simulink model "nxtracer"  (Simulink 6.4)
settings: Solver=ode4  StartTime=0.0  StopTime=inf  FixedStep=Ts  RelTol=1e-3
PreLoadFcn:
  | param;
values from neighbouring files (symbols this model uses):
  CAMERA_POS = [100 100]    [param.m]
  Cm = 9.00e-6    (= 9e-06)    [param.m]
  Cw = 9.00e-4    (= 0.0009)    [param.m]
  Dx = 1e-3    (= 0.001)    [param.m]
  Dzz = 1e-6    (= 1e-06)    [param.m]
  e = -0.2    [param.m]
  J = M*(W/2)^2    (= 0.004096)    [param.m]
  Jm = 0.5e-7    (= 5e-08)    [param.m]
  Jw = 20.0e-7    (= 2e-06)    [param.m]
  Kb = 0.022    [param.m]
  Kt = 0.022    [param.m]
  LENGTH = 20    [param.m]
  LENGTH1 = 12    [param.m]
  LENGTH2 = 16    [param.m]
  LINE_MAP = ~(TRACK_MAP - LINE)    [param.m]
  Lm = 1.4e-3    (= 0.0014)    [param.m]
  M = 0.64    [param.m]
  n = 24    [param.m]
  Rm = 1.0    (= 1)    [param.m]
  Rw = 0.056/2    (= 0.028)    [param.m]
  START_POS = [148 100]    [param.m]
  TRACK_MAP = double(imread('track.bmp'))    [param.m]
  Ts = 0.0001    [param.m]
  W = 0.16    [param.m]
  WALL_MAP = ~(TRACK_MAP - WALL)    [param.m]
  WIDTH = 16    [param.m]
  WIDTH1 = 12    [param.m]
undefined symbols (not defined in the file or in its folder): clearNXTSignalObjects, DiscIntNeverNeededParam
libraries: simulink x12, vrlib x1, ecrobot_nxt_lib x1
(part 2 of 3)

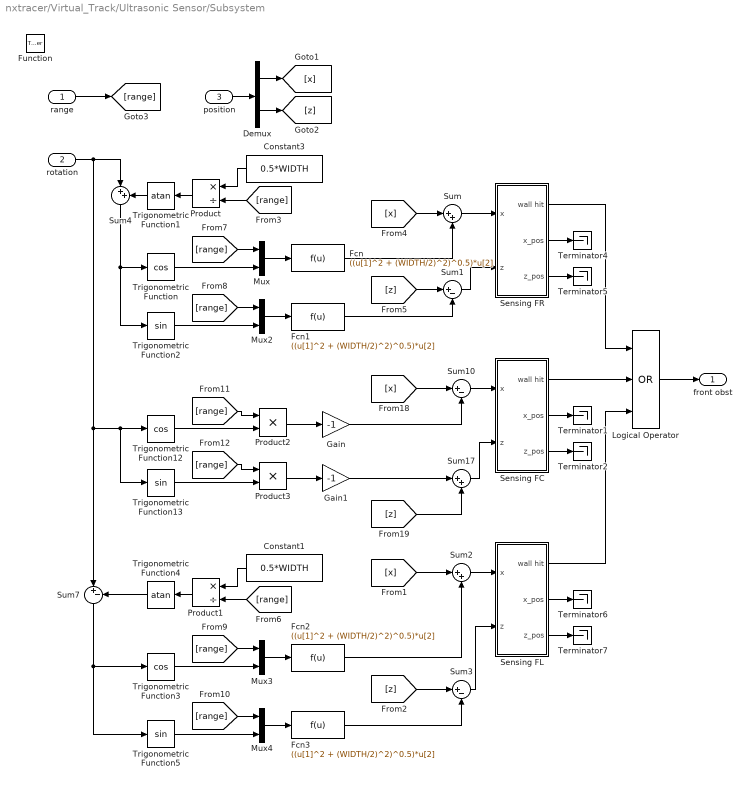
== system nxtracer/Virtual_Track/Ultrasonic Sensor/Subsystem ==
  range : Inport
  rotation : Inport  Port=2
  position : Inport  Port=3
  Function : TriggerPort  TriggerType=function-call
  Constant1 : Constant  Orientation=left  Value=0.5*WIDTH  OutDataType=sfix(16)  ConRadixGroup=Use specified scaling  OutScaling=2^0  SampleTime=inf  FramePeriod=inf
  Constant3 : Constant  Orientation=left  Value=0.5*WIDTH  OutDataType=sfix(16)  ConRadixGroup=Use specified scaling  OutScaling=2^0  SampleTime=inf  FramePeriod=inf
  Demux : Demux  Outputs=2
  Fcn{,1..3} (4 alike) : Fcn  Expr=((u[1]^2 + (WIDTH/2)^2)^0.5)*u[2]
  Gain : Gain  Gain=-1
  Gain1 : Gain  Gain=-1
  Logical Operator : Logic  Operator=OR  Inputs=3  AllPortsSameDT=off  OutDataTypeMode=Boolean
  Mux{,2..4} (4 alike) : Mux  Inputs=2
  Product : Product  Orientation=left  Inputs=*/  RndMeth=Zero
  Product1 : Product  Orientation=left  Inputs=*/  RndMeth=Zero
  Product2 : Product  RndMeth=Zero
  Product3 : Product  RndMeth=Zero
  Sensing FC : Subsystem
  Sensing FL : Subsystem
  Sensing FR : Subsystem
  Sum : Sum  Inputs=|++
  Sum1 : Sum  Inputs=|+-
  Sum10 : Sum  Inputs=|+-
  Sum17 : Sum  Inputs=|++
  Sum2 : Sum  Inputs=|++
  Sum3 : Sum  Inputs=|+-
  Sum4 : Sum  Orientation=down  Inputs=|++
  Sum7 : Sum  Orientation=down  Inputs=|+-
  Terminator{1..2,4..7} (6 alike) : Terminator
  Trigonometric Function : Trigonometry  Operator=cos
  Trigonometric Function1 : Trigonometry  Orientation=left  Operator=atan
  Trigonometric Function12 : Trigonometry  Operator=cos
  Trigonometric Function13 : Trigonometry
  Trigonometric Function2 : Trigonometry
  Trigonometric Function3 : Trigonometry  Operator=cos
  Trigonometric Function4 : Trigonometry  Orientation=left  Operator=atan
  Trigonometric Function5 : Trigonometry
  front obst : Outport  InitialOutput=0
  wires:
  Sensing FC/3(z_pos) -> Terminator2/1
  Sensing FL/1(wall hit) -> Logical Operator/3
  [z] -> Sum17/2
  [x] -> Sum10/1
  Sum10/1 -> Sensing FC/1(x)
  Product3/1 -> Gain1/1
  Sum17/1 -> Sensing FC/2(z)
  Trigonometric Function12/1 -> Product2/2
  Product2/1 -> Gain/1
  Trigonometric Function13/1 -> Product3/2
  Sensing FC/1(wall hit) -> Logical Operator/2
  Sensing FC/2(x_pos) -> Terminator1/1
  Sensing FR/3(z_pos) -> Terminator5/1
  Sum3/1 -> Sensing FL/2(z)
  Trigonometric Function1/1 -> Sum4/2
  Product/1 -> Trigonometric Function1/1
  Sensing FR/1(wall hit) -> Logical Operator/1
  Sensing FR/2(x_pos) -> Terminator4/1
  Sensing FL/2(x_pos) -> Terminator6/1
  Sensing FL/3(z_pos) -> Terminator7/1
  Sum/1 -> Sensing FR/1(x)
  [z] -> Sum1/1
  [x] -> Sum/1
  Trigonometric Function/1 -> Mux/2
  Sum1/1 -> Sensing FR/2(z)
  Sum4/1 -> Trigonometric Function2/1, Trigonometric Function/1
  Fcn1/1 -> Sum1/2
  Sum2/1 -> Sensing FL/1(x)
  [z] -> Sum3/1
  [x] -> Sum2/1
  Trigonometric Function3/1 -> Mux3/2
  Sum7/1 -> Trigonometric Function5/1, Trigonometric Function3/1
  Trigonometric Function4/1 -> Sum7/2
  Fcn3/1 -> Sum3/2
  Fcn2/1 -> Sum2/2
  rotation/1 -> Trigonometric Function13/1, Trigonometric Function12/1, Sum7/1, Sum4/1
  Demux/2 -> [z]
  Demux/1 -> [x]
  position/1 -> Demux/1
  range/1 -> [range]
  [range] -> Product/2
  Constant3/1 -> Product/1
  [range] -> Product1/2
  Constant1/1 -> Product1/1
  Product1/1 -> Trigonometric Function4/1
  [range] -> Mux/1
  Mux/1 -> Fcn/1
  Fcn/1 -> Sum/2
  [range] -> Mux2/1
  Mux2/1 -> Fcn1/1
  Trigonometric Function2/1 -> Mux2/2
  [range] -> Mux3/1
  Mux3/1 -> Fcn2/1
  Trigonometric Function5/1 -> Mux4/2
  [range] -> Mux4/1
  Mux4/1 -> Fcn3/1
  [range] -> Product2/1
  Gain/1 -> Sum10/2
  [range] -> Product3/1
  Gain1/1 -> Sum17/1
  Logical Operator/1 -> front obst/1

== system nxtracer/Virtual_Track/Virtual Reality/ calc camera pos ==
  x : Inport
  z : Inport  Port=2
  rot : Inport  Port=3
  Mux3 : Mux  Inputs=3
  Terminator : Terminator
  y1 : Constant  Value=7  OutDataType=sfix(16)  ConRadixGroup=Use specified scaling  OutScaling=2^0  SampleTime=inf  FramePeriod=inf
  Out1 : Outport
  wires:
  y1/1 -> Mux3/2
  Mux3/1 -> Out1/1
  z/1 -> Mux3/3
  x/1 -> Mux3/1
  rot/1 -> Terminator/1

== system nxtracer/Virtual_Track/Virtual Reality/calc camera rot ==
  x : Inport
  z : Inport  Port=2
  Abs : Abs  SampleTime=-1  SaturateOnIntegerOverflow=off
  Backlash : Backlash  BacklashWidth=8
  Backlash2 : Backlash  BacklashWidth=8
  If : If  NumInputs=2  IfExpression=u1>0 & u2<=0  ElseIfExpressions=u1<=0 & u2<=0, u1<=0 & u2>0
  If Action Subsystem : Subsystem  TreatAsAtomicUnit=on
  If Action Subsystem1 : Subsystem  TreatAsAtomicUnit=on
  If Action Subsystem2 : Subsystem  TreatAsAtomicUnit=on
  If Action Subsystem3 : Subsystem  TreatAsAtomicUnit=on
  Merge : Merge  Inputs=4
  Mux3 : Mux  Inputs=2
  Product : Product  Inputs=*/  RndMeth=Zero
  Sum : Sum  Inputs=|+-
  Sum1 : Sum  Inputs=|+-
  Trigonometric Function : Trigonometry  Operator=atan
  relative pos x : Constant  Value=CAMERA_POS(2)-100  OutDataType=sfix(16)  ConRadixGroup=Use specified scaling  OutScaling=2^0  SampleTime=inf  FramePeriod=inf
  relative pos x1 : Constant  Value=100-CAMERA_POS(1)  OutDataType=sfix(16)  ConRadixGroup=Use specified scaling  OutScaling=2^0  SampleTime=inf  FramePeriod=inf
  rotation_x_y_z : Constant  Value=[0 1 0]  OutDataType=sfix(16)  ConRadixGroup=Use specified scaling  OutScaling=2^0  SampleTime=inf  FramePeriod=inf
  rot : Outport
  wires:
  x/1 -> Backlash/1
  relative pos x/1 -> Sum/1
  Backlash/1 -> Sum/2
  Backlash2/1 -> Sum1/2
  z/1 -> Backlash2/1
  Sum/1 -> Product/1, If/1
  Sum1/1 -> Product/2, If/2
  Product/1 -> Abs/1
  Abs/1 -> Trigonometric Function/1
  If/1 -> If Action Subsystem/Action
  If/2 -> If Action Subsystem1/Action
  If/3 -> If Action Subsystem2/Action
  If/4 -> If Action Subsystem3/Action
  Trigonometric Function/1 -> [rot]
  [rot] -> If Action Subsystem/1(In1)
  [rot] -> If Action Subsystem1/1(In1)
  [rot] -> If Action Subsystem2/1(In1)
  [rot] -> If Action Subsystem3/1(In1)
  If Action Subsystem/1(Out1) -> Merge/1
  If Action Subsystem1/1(Out1) -> Merge/2
  If Action Subsystem2/1(Out1) -> Merge/3
  If Action Subsystem3/1(Out1) -> Merge/4
  Merge/1 -> Mux3/2
  relative pos x1/1 -> Sum1/1
  Mux3/1 -> rot/1
  rotation_x_y_z/1 -> Mux3/1

== system nxtracer/Virtual_Track/Virtual Reality/calc rear tyre assy rot ==
  rot : Inport
  speed : Inport  Port=2
  tyre rot speed : Inport  Port=3
  wall hit : Inport  Port=4
  calc rear tyre hub rot : Subsystem
  calc rear tyre rev : Subsystem
  rear hub rot : Outport
  rear tyre rot : Outport  Port=2
  wires:
  speed/1 -> calc rear tyre rev/3(speed), calc rear tyre hub rot/2(speed)
  calc rear tyre hub rot/2(Out2) -> calc rear tyre rev/1(spin_flag)
  rot/1 -> calc rear tyre hub rot/1(rot)
  calc rear tyre hub rot/1(Out1) -> rear hub rot/1
  calc rear tyre rev/1(Out1) -> rear tyre rot/1
  tyre rot speed/1 -> calc rear tyre rev/2(tyre rotSpeed)
  wall hit/1 -> calc rear tyre rev/4(wall hit)

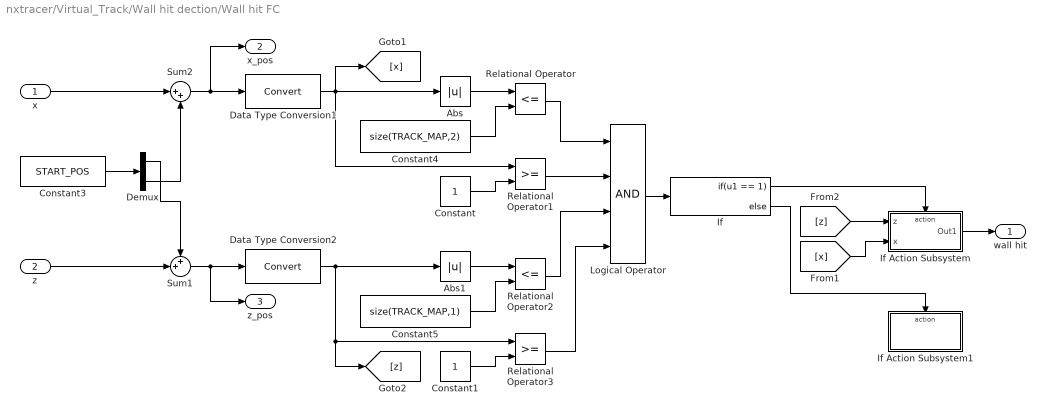
== system nxtracer/Virtual_Track/Wall hit dection/Wall hit FC ==
  x : Inport
  z : Inport  Port=2
  Abs : Abs  SampleTime=-1  SaturateOnIntegerOverflow=off
  Abs1 : Abs  SampleTime=-1  SaturateOnIntegerOverflow=off
  Constant : Constant  Value=1  OutDataType=sfix(16)  ConRadixGroup=Use specified scaling  OutScaling=2^0  SampleTime=inf  FramePeriod=inf
  Constant1 : Constant  Value=1  OutDataType=sfix(16)  ConRadixGroup=Use specified scaling  OutScaling=2^0  SampleTime=inf  FramePeriod=inf
  Constant3 : Constant  Value=START_POS  OutDataType=sfix(16)  ConRadixGroup=Use specified scaling  OutScaling=2^0  SampleTime=inf  FramePeriod=inf
  Constant4 : Constant  Value=size(TRACK_MAP,2)  OutDataType=sfix(16)  ConRadixGroup=Use specified scaling  OutScaling=2^0  SampleTime=inf  FramePeriod=inf
  Constant5 : Constant  Value=size(TRACK_MAP,1)  OutDataType=sfix(16)  ConRadixGroup=Use specified scaling  OutScaling=2^0  SampleTime=inf  FramePeriod=inf
  Data Type Conversion1 : DataTypeConversion  OutDataTypeMode=uint32  SaturateOnIntegerOverflow=on
  Data Type Conversion2 : DataTypeConversion  OutDataTypeMode=uint32  SaturateOnIntegerOverflow=on
  Demux : Demux  Outputs=2
  If : If  IfExpression=u1 == 1
  If Action Subsystem : Subsystem  TreatAsAtomicUnit=on
  If Action Subsystem1 : Subsystem  TreatAsAtomicUnit=on
  Logical Operator : Logic  Inputs=4  AllPortsSameDT=off  OutDataTypeMode=Boolean
  Relational Operator : RelationalOperator  Operator=<=  LogicOutDataTypeMode=Boolean
  Relational Operator1 : RelationalOperator  LogicOutDataTypeMode=Boolean
  Relational Operator2 : RelationalOperator  Operator=<=  LogicOutDataTypeMode=Boolean
  Relational Operator3 : RelationalOperator  LogicOutDataTypeMode=Boolean
  Sum1 : Sum  Inputs=++|
  Sum2 : Sum  Inputs=|++
  wall hit : Outport
  x_pos : Outport  Port=2
  z_pos : Outport  Port=3
  wires:
  [x] -> If Action Subsystem/2(x)
  [z] -> If Action Subsystem/1(z)
  Data Type Conversion1/1 -> [x], Relational Operator1/1, Abs/1
  Data Type Conversion2/1 -> [z], Relational Operator3/1, Abs1/1
  Sum2/1 -> x_pos/1, Data Type Conversion1/1
  If Action Subsystem/1(Out1) -> wall hit/1
  If/2 -> If Action Subsystem1/Action
  If/1 -> If Action Subsystem/Action
  Relational Operator1/1 -> Logical Operator/2
  Logical Operator/1 -> If/1
  Relational Operator3/1 -> Logical Operator/4
  Relational Operator2/1 -> Logical Operator/3
  Relational Operator/1 -> Logical Operator/1
  Constant1/1 -> Relational Operator3/2
  Constant5/1 -> Relational Operator2/2
  Abs1/1 -> Relational Operator2/1
  Constant/1 -> Relational Operator1/2
  Constant4/1 -> Relational Operator/2
  Abs/1 -> Relational Operator/1
  Sum1/1 -> z_pos/1, Data Type Conversion2/1
  z/1 -> Sum1/2
  Demux/1 -> Sum1/1
  x/1 -> Sum2/1
  Demux/2 -> Sum2/2
  Constant3/1 -> Demux/1

== system nxtracer/Virtual_Track/Wall hit dection/Wall hit FL ==
  x : Inport
  z : Inport  Port=2
  Abs : Abs  SampleTime=-1  SaturateOnIntegerOverflow=off
  Abs1 : Abs  SampleTime=-1  SaturateOnIntegerOverflow=off
  Constant : Constant  Value=1  OutDataType=sfix(16)  ConRadixGroup=Use specified scaling  OutScaling=2^0  SampleTime=inf  FramePeriod=inf
  Constant1 : Constant  Value=1  OutDataType=sfix(16)  ConRadixGroup=Use specified scaling  OutScaling=2^0  SampleTime=inf  FramePeriod=inf
  Constant3 : Constant  Value=START_POS  OutDataType=sfix(16)  ConRadixGroup=Use specified scaling  OutScaling=2^0  SampleTime=inf  FramePeriod=inf
  Constant4 : Constant  Value=size(TRACK_MAP,2)  OutDataType=sfix(16)  ConRadixGroup=Use specified scaling  OutScaling=2^0  SampleTime=inf  FramePeriod=inf
  Constant5 : Constant  Value=size(TRACK_MAP,1)  OutDataType=sfix(16)  ConRadixGroup=Use specified scaling  OutScaling=2^0  SampleTime=inf  FramePeriod=inf
  Data Type Conversion1 : DataTypeConversion  OutDataTypeMode=uint32  SaturateOnIntegerOverflow=on
  Data Type Conversion2 : DataTypeConversion  OutDataTypeMode=uint32  SaturateOnIntegerOverflow=on
  Demux : Demux  Outputs=2
  If : If  IfExpression=u1 == 1
  If Action Subsystem : Subsystem  TreatAsAtomicUnit=on
  If Action Subsystem1 : Subsystem  TreatAsAtomicUnit=on
  Logical Operator : Logic  Inputs=4  AllPortsSameDT=off  OutDataTypeMode=Boolean
  Relational Operator : RelationalOperator  Operator=<=  LogicOutDataTypeMode=Boolean
  Relational Operator1 : RelationalOperator  LogicOutDataTypeMode=Boolean
  Relational Operator2 : RelationalOperator  Operator=<=  LogicOutDataTypeMode=Boolean
  Relational Operator3 : RelationalOperator  LogicOutDataTypeMode=Boolean
  Sum1 : Sum  Inputs=++|
  Sum2 : Sum  Inputs=|++
  wall hit : Outport
  x_pos : Outport  Port=2
  z_pos : Outport  Port=3
  wires:
  Constant3/1 -> Demux/1
  Demux/2 -> Sum2/2
  x/1 -> Sum2/1
  Demux/1 -> Sum1/1
  z/1 -> Sum1/2
  Sum1/1 -> Data Type Conversion2/1, z_pos/1
  Abs/1 -> Relational Operator/1
  Constant4/1 -> Relational Operator/2
  Constant/1 -> Relational Operator1/2
  Abs1/1 -> Relational Operator2/1
  Constant5/1 -> Relational Operator2/2
  Constant1/1 -> Relational Operator3/2
  Relational Operator/1 -> Logical Operator/1
  Relational Operator2/1 -> Logical Operator/3
  Relational Operator3/1 -> Logical Operator/4
  Logical Operator/1 -> If/1
  Relational Operator1/1 -> Logical Operator/2
  If/1 -> If Action Subsystem/Action
  If/2 -> If Action Subsystem1/Action
  If Action Subsystem/1(Out1) -> wall hit/1
  Sum2/1 -> Data Type Conversion1/1, x_pos/1
  Data Type Conversion2/1 -> Abs1/1, Relational Operator3/1, [z]
  Data Type Conversion1/1 -> Abs/1, Relational Operator1/1, [x]
  [z] -> If Action Subsystem/1(z)
  [x] -> If Action Subsystem/2(x)

== system nxtracer/Virtual_Track/Wall hit dection/Wall hit FR ==
  x : Inport
  z : Inport  Port=2
  Abs : Abs  SampleTime=-1  SaturateOnIntegerOverflow=off
  Abs1 : Abs  SampleTime=-1  SaturateOnIntegerOverflow=off
  Constant : Constant  Value=1  OutDataType=sfix(16)  ConRadixGroup=Use specified scaling  OutScaling=2^0  SampleTime=inf  FramePeriod=inf
  Constant1 : Constant  Value=1  OutDataType=sfix(16)  ConRadixGroup=Use specified scaling  OutScaling=2^0  SampleTime=inf  FramePeriod=inf
  Constant3 : Constant  Value=START_POS  OutDataType=sfix(16)  ConRadixGroup=Use specified scaling  OutScaling=2^0  SampleTime=inf  FramePeriod=inf
  Constant4 : Constant  Value=size(TRACK_MAP,2)  OutDataType=sfix(16)  ConRadixGroup=Use specified scaling  OutScaling=2^0  SampleTime=inf  FramePeriod=inf
  Constant5 : Constant  Value=size(TRACK_MAP,1)  OutDataType=sfix(16)  ConRadixGroup=Use specified scaling  OutScaling=2^0  SampleTime=inf  FramePeriod=inf
  Data Type Conversion1 : DataTypeConversion  OutDataTypeMode=uint32  SaturateOnIntegerOverflow=on
  Data Type Conversion2 : DataTypeConversion  OutDataTypeMode=uint32  SaturateOnIntegerOverflow=on
  Demux : Demux  Outputs=2
  If : If  IfExpression=u1 == 1
  If Action Subsystem : Subsystem  TreatAsAtomicUnit=on
  If Action Subsystem1 : Subsystem  TreatAsAtomicUnit=on
  Logical Operator : Logic  Inputs=4  AllPortsSameDT=off  OutDataTypeMode=Boolean
  Relational Operator : RelationalOperator  Operator=<=  LogicOutDataTypeMode=Boolean
  Relational Operator1 : RelationalOperator  LogicOutDataTypeMode=Boolean
  Relational Operator2 : RelationalOperator  Operator=<=  LogicOutDataTypeMode=Boolean
  Relational Operator3 : RelationalOperator  LogicOutDataTypeMode=Boolean
  Sum1 : Sum  Inputs=++|
  Sum2 : Sum  Inputs=|++
  wall hit : Outport
  x_pos : Outport  Port=2
  z_pos : Outport  Port=3
  wires:
  Constant3/1 -> Demux/1
  Demux/2 -> Sum2/2
  x/1 -> Sum2/1
  Demux/1 -> Sum1/1
  z/1 -> Sum1/2
  Sum1/1 -> Data Type Conversion2/1, z_pos/1
  Abs/1 -> Relational Operator/1
  Constant4/1 -> Relational Operator/2
  Constant/1 -> Relational Operator1/2
  Abs1/1 -> Relational Operator2/1
  Constant5/1 -> Relational Operator2/2
  Constant1/1 -> Relational Operator3/2
  Relational Operator/1 -> Logical Operator/1
  Relational Operator2/1 -> Logical Operator/3
  Relational Operator3/1 -> Logical Operator/4
  Logical Operator/1 -> If/1
  Relational Operator1/1 -> Logical Operator/2
  If/1 -> If Action Subsystem/Action
  If/2 -> If Action Subsystem1/Action
  If Action Subsystem/1(Out1) -> wall hit/1
  Sum2/1 -> Data Type Conversion1/1, x_pos/1
  Data Type Conversion2/1 -> Abs1/1, Relational Operator3/1, [z]
  Data Type Conversion1/1 -> Abs/1, Relational Operator1/1, [x]
  [z] -> If Action Subsystem/1(z)
  [x] -> If Action Subsystem/2(x)

== system nxtracer/Virtual_Track/Wall hit dection/Wall hit RC ==
  x : Inport
  z : Inport  Port=2
  Abs : Abs  SampleTime=-1  SaturateOnIntegerOverflow=off
  Abs1 : Abs  SampleTime=-1  SaturateOnIntegerOverflow=off
  Constant : Constant  Value=1  OutDataType=sfix(16)  ConRadixGroup=Use specified scaling  OutScaling=2^0  SampleTime=inf  FramePeriod=inf
  Constant1 : Constant  Value=1  OutDataType=sfix(16)  ConRadixGroup=Use specified scaling  OutScaling=2^0  SampleTime=inf  FramePeriod=inf
  Constant3 : Constant  Value=START_POS  OutDataType=sfix(16)  ConRadixGroup=Use specified scaling  OutScaling=2^0  SampleTime=inf  FramePeriod=inf
  Constant4 : Constant  Value=size(TRACK_MAP,2)  OutDataType=sfix(16)  ConRadixGroup=Use specified scaling  OutScaling=2^0  SampleTime=inf  FramePeriod=inf
  Constant5 : Constant  Value=size(TRACK_MAP,1)  OutDataType=sfix(16)  ConRadixGroup=Use specified scaling  OutScaling=2^0  SampleTime=inf  FramePeriod=inf
  Data Type Conversion1 : DataTypeConversion  OutDataTypeMode=uint32  SaturateOnIntegerOverflow=on
  Data Type Conversion2 : DataTypeConversion  OutDataTypeMode=uint32  SaturateOnIntegerOverflow=on
  Demux : Demux  Outputs=2
  If : If  IfExpression=u1 == 1
  If Action Subsystem : Subsystem  TreatAsAtomicUnit=on
  If Action Subsystem1 : Subsystem  TreatAsAtomicUnit=on
  Logical Operator : Logic  Inputs=4  AllPortsSameDT=off  OutDataTypeMode=Boolean
  Relational Operator : RelationalOperator  Operator=<=  LogicOutDataTypeMode=Boolean
  Relational Operator1 : RelationalOperator  LogicOutDataTypeMode=Boolean
  Relational Operator2 : RelationalOperator  Operator=<=  LogicOutDataTypeMode=Boolean
  Relational Operator3 : RelationalOperator  LogicOutDataTypeMode=Boolean
  Sum1 : Sum  Inputs=++|
  Sum2 : Sum  Inputs=|++
  wall hit : Outport
  x_pos : Outport  Port=2
  z_pos : Outport  Port=3
  wires:
  Constant3/1 -> Demux/1
  Demux/2 -> Sum2/2
  x/1 -> Sum2/1
  Demux/1 -> Sum1/1
  z/1 -> Sum1/2
  Sum1/1 -> Data Type Conversion2/1, z_pos/1
  Abs/1 -> Relational Operator/1
  Constant4/1 -> Relational Operator/2
  Constant/1 -> Relational Operator1/2
  Abs1/1 -> Relational Operator2/1
  Constant5/1 -> Relational Operator2/2
  Constant1/1 -> Relational Operator3/2
  Relational Operator/1 -> Logical Operator/1
  Relational Operator2/1 -> Logical Operator/3
  Relational Operator3/1 -> Logical Operator/4
  Logical Operator/1 -> If/1
  Relational Operator1/1 -> Logical Operator/2
  If/1 -> If Action Subsystem/Action
  If/2 -> If Action Subsystem1/Action
  If Action Subsystem/1(Out1) -> wall hit/1
  Sum2/1 -> Data Type Conversion1/1, x_pos/1
  Data Type Conversion2/1 -> Abs1/1, Relational Operator3/1, [z]
  Data Type Conversion1/1 -> Abs/1, Relational Operator1/1, [x]
  [z] -> If Action Subsystem/1(z)
  [x] -> If Action Subsystem/2(x)

== system nxtracer/Virtual_Track/Wall hit dection/Wall hit RL ==
  x : Inport
  z : Inport  Port=2
  Abs : Abs  SampleTime=-1  SaturateOnIntegerOverflow=off
  Abs1 : Abs  SampleTime=-1  SaturateOnIntegerOverflow=off
  Constant : Constant  Value=1  OutDataType=sfix(16)  ConRadixGroup=Use specified scaling  OutScaling=2^0  SampleTime=inf  FramePeriod=inf
  Constant1 : Constant  Value=1  OutDataType=sfix(16)  ConRadixGroup=Use specified scaling  OutScaling=2^0  SampleTime=inf  FramePeriod=inf
  Constant3 : Constant  Value=START_POS  OutDataType=sfix(16)  ConRadixGroup=Use specified scaling  OutScaling=2^0  SampleTime=inf  FramePeriod=inf
  Constant4 : Constant  Value=size(TRACK_MAP,2)  OutDataType=sfix(16)  ConRadixGroup=Use specified scaling  OutScaling=2^0  SampleTime=inf  FramePeriod=inf
  Constant5 : Constant  Value=size(TRACK_MAP,1)  OutDataType=sfix(16)  ConRadixGroup=Use specified scaling  OutScaling=2^0  SampleTime=inf  FramePeriod=inf
  Data Type Conversion1 : DataTypeConversion  OutDataTypeMode=uint32  SaturateOnIntegerOverflow=on
  Data Type Conversion2 : DataTypeConversion  OutDataTypeMode=uint32  SaturateOnIntegerOverflow=on
  Demux : Demux  Outputs=2
  If : If  IfExpression=u1 == 1
  If Action Subsystem : Subsystem  TreatAsAtomicUnit=on
  If Action Subsystem1 : Subsystem  TreatAsAtomicUnit=on
  Logical Operator : Logic  Inputs=4  AllPortsSameDT=off  OutDataTypeMode=Boolean
  Relational Operator : RelationalOperator  Operator=<=  LogicOutDataTypeMode=Boolean
  Relational Operator1 : RelationalOperator  LogicOutDataTypeMode=Boolean
  Relational Operator2 : RelationalOperator  Operator=<=  LogicOutDataTypeMode=Boolean
  Relational Operator3 : RelationalOperator  LogicOutDataTypeMode=Boolean
  Sum1 : Sum  Inputs=++|
  Sum2 : Sum  Inputs=|++
  wall hit : Outport
  x_pos : Outport  Port=2
  z_pos : Outport  Port=3
  wires:
  Constant3/1 -> Demux/1
  Demux/2 -> Sum2/2
  x/1 -> Sum2/1
  Demux/1 -> Sum1/1
  z/1 -> Sum1/2
  Sum1/1 -> Data Type Conversion2/1, z_pos/1
  Abs/1 -> Relational Operator/1
  Constant4/1 -> Relational Operator/2
  Constant/1 -> Relational Operator1/2
  Abs1/1 -> Relational Operator2/1
  Constant5/1 -> Relational Operator2/2
  Constant1/1 -> Relational Operator3/2
  Relational Operator/1 -> Logical Operator/1
  Relational Operator2/1 -> Logical Operator/3
  Relational Operator3/1 -> Logical Operator/4
  Logical Operator/1 -> If/1
  Relational Operator1/1 -> Logical Operator/2
  If/1 -> If Action Subsystem/Action
  If/2 -> If Action Subsystem1/Action
  If Action Subsystem/1(Out1) -> wall hit/1
  Sum2/1 -> Data Type Conversion1/1, x_pos/1
  Data Type Conversion2/1 -> Abs1/1, Relational Operator3/1, [z]
  Data Type Conversion1/1 -> Abs/1, Relational Operator1/1, [x]
  [z] -> If Action Subsystem/1(z)
  [x] -> If Action Subsystem/2(x)

== system nxtracer/Virtual_Track/Wall hit dection/Wall hit RR ==
  x : Inport
  z : Inport  Port=2
  Abs : Abs  SampleTime=-1  SaturateOnIntegerOverflow=off
  Abs1 : Abs  SampleTime=-1  SaturateOnIntegerOverflow=off
  Constant : Constant  Value=1  OutDataType=sfix(16)  ConRadixGroup=Use specified scaling  OutScaling=2^0  SampleTime=inf  FramePeriod=inf
  Constant1 : Constant  Value=1  OutDataType=sfix(16)  ConRadixGroup=Use specified scaling  OutScaling=2^0  SampleTime=inf  FramePeriod=inf
  Constant3 : Constant  Value=START_POS  OutDataType=sfix(16)  ConRadixGroup=Use specified scaling  OutScaling=2^0  SampleTime=inf  FramePeriod=inf
  Constant4 : Constant  Value=size(TRACK_MAP,2)  OutDataType=sfix(16)  ConRadixGroup=Use specified scaling  OutScaling=2^0  SampleTime=inf  FramePeriod=inf
  Constant5 : Constant  Value=size(TRACK_MAP,1)  OutDataType=sfix(16)  ConRadixGroup=Use specified scaling  OutScaling=2^0  SampleTime=inf  FramePeriod=inf
  Data Type Conversion1 : DataTypeConversion  OutDataTypeMode=uint32  SaturateOnIntegerOverflow=on
  Data Type Conversion2 : DataTypeConversion  OutDataTypeMode=uint32  SaturateOnIntegerOverflow=on
  Demux : Demux  Outputs=2
  If : If  IfExpression=u1 == 1
  If Action Subsystem : Subsystem  TreatAsAtomicUnit=on
  If Action Subsystem1 : Subsystem  TreatAsAtomicUnit=on
  Logical Operator : Logic  Inputs=4  AllPortsSameDT=off  OutDataTypeMode=Boolean
  Relational Operator : RelationalOperator  Operator=<=  LogicOutDataTypeMode=Boolean
  Relational Operator1 : RelationalOperator  LogicOutDataTypeMode=Boolean
  Relational Operator2 : RelationalOperator  Operator=<=  LogicOutDataTypeMode=Boolean
  Relational Operator3 : RelationalOperator  LogicOutDataTypeMode=Boolean
  Sum1 : Sum  Inputs=++|
  Sum2 : Sum  Inputs=|++
  wall hit : Outport
  x_pos : Outport  Port=2
  z_pos : Outport  Port=3
  wires:
  [x] -> If Action Subsystem/2(x)
  [z] -> If Action Subsystem/1(z)
  Data Type Conversion1/1 -> [x], Relational Operator1/1, Abs/1
  Data Type Conversion2/1 -> [z], Relational Operator3/1, Abs1/1
  Sum2/1 -> x_pos/1, Data Type Conversion1/1
  If Action Subsystem/1(Out1) -> wall hit/1
  If/2 -> If Action Subsystem1/Action
  If/1 -> If Action Subsystem/Action
  Relational Operator1/1 -> Logical Operator/2
  Logical Operator/1 -> If/1
  Relational Operator3/1 -> Logical Operator/4
  Relational Operator2/1 -> Logical Operator/3
  Relational Operator/1 -> Logical Operator/1
  Constant1/1 -> Relational Operator3/2
  Constant5/1 -> Relational Operator2/2
  Abs1/1 -> Relational Operator2/1
  Constant/1 -> Relational Operator1/2
  Constant4/1 -> Relational Operator/2
  Abs/1 -> Relational Operator/1
  Sum1/1 -> z_pos/1, Data Type Conversion2/1
  z/1 -> Sum1/2
  Demux/1 -> Sum1/1
  x/1 -> Sum2/1
  Demux/2 -> Sum2/2
  Constant3/1 -> Demux/1

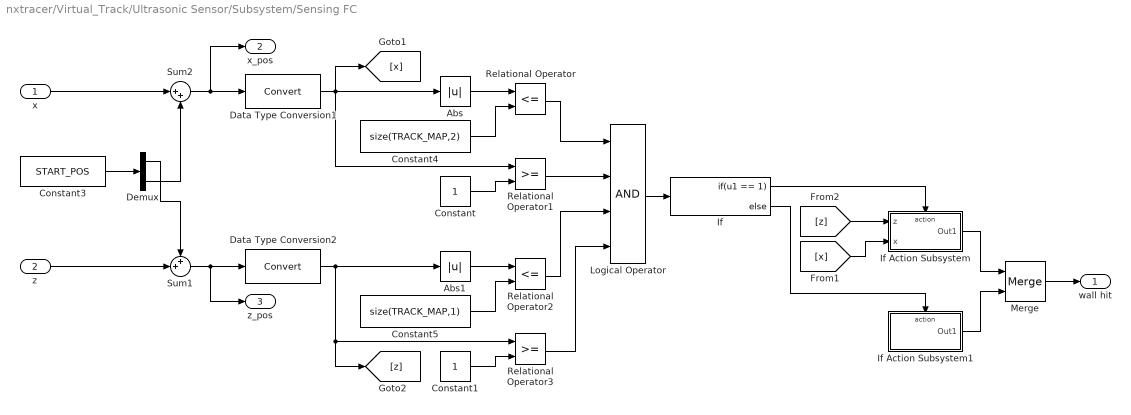
== system nxtracer/Virtual_Track/Ultrasonic Sensor/Subsystem/Sensing FC ==
  x : Inport
  z : Inport  Port=2
  Abs : Abs  SampleTime=-1  SaturateOnIntegerOverflow=off
  Abs1 : Abs  SampleTime=-1  SaturateOnIntegerOverflow=off
  Constant : Constant  Value=1  OutDataType=sfix(16)  ConRadixGroup=Use specified scaling  OutScaling=2^0  SampleTime=inf  FramePeriod=inf
  Constant1 : Constant  Value=1  OutDataType=sfix(16)  ConRadixGroup=Use specified scaling  OutScaling=2^0  SampleTime=inf  FramePeriod=inf
  Constant3 : Constant  Value=START_POS  OutDataType=sfix(16)  ConRadixGroup=Use specified scaling  OutScaling=2^0  SampleTime=inf  FramePeriod=inf
  Constant4 : Constant  Value=size(TRACK_MAP,2)  OutDataType=sfix(16)  ConRadixGroup=Use specified scaling  OutScaling=2^0  SampleTime=inf  FramePeriod=inf
  Constant5 : Constant  Value=size(TRACK_MAP,1)  OutDataType=sfix(16)  ConRadixGroup=Use specified scaling  OutScaling=2^0  SampleTime=inf  FramePeriod=inf
  Data Type Conversion1 : DataTypeConversion  OutDataTypeMode=int32  SaturateOnIntegerOverflow=on
  Data Type Conversion2 : DataTypeConversion  OutDataTypeMode=int32  SaturateOnIntegerOverflow=on
  Demux : Demux  Outputs=2
  If : If  IfExpression=u1 == 1
  If Action Subsystem : Subsystem  TreatAsAtomicUnit=on
  If Action Subsystem1 : Subsystem  TreatAsAtomicUnit=on
  Logical Operator : Logic  Inputs=4  AllPortsSameDT=off  OutDataTypeMode=Boolean
  Merge : Merge
  Relational Operator : RelationalOperator  Operator=<=  LogicOutDataTypeMode=Boolean
  Relational Operator1 : RelationalOperator  LogicOutDataTypeMode=Boolean
  Relational Operator2 : RelationalOperator  Operator=<=  LogicOutDataTypeMode=Boolean
  Relational Operator3 : RelationalOperator  LogicOutDataTypeMode=Boolean
  Sum1 : Sum  Inputs=++|
  Sum2 : Sum  Inputs=|++
  wall hit : Outport
  x_pos : Outport  Port=2
  z_pos : Outport  Port=3
  wires:
  Merge/1 -> wall hit/1
  If Action Subsystem1/1(Out1) -> Merge/2
  If Action Subsystem/1(Out1) -> Merge/1
  [x] -> If Action Subsystem/2(x)
  [z] -> If Action Subsystem/1(z)
  Data Type Conversion1/1 -> [x], Relational Operator1/1, Abs/1
  Data Type Conversion2/1 -> [z], Relational Operator3/1, Abs1/1
  Sum2/1 -> x_pos/1, Data Type Conversion1/1
  If/2 -> If Action Subsystem1/Action
  If/1 -> If Action Subsystem/Action
  Relational Operator1/1 -> Logical Operator/2
  Logical Operator/1 -> If/1
  Relational Operator3/1 -> Logical Operator/4
  Relational Operator2/1 -> Logical Operator/3
  Relational Operator/1 -> Logical Operator/1
  Constant1/1 -> Relational Operator3/2
  Constant5/1 -> Relational Operator2/2
  Abs1/1 -> Relational Operator2/1
  Constant/1 -> Relational Operator1/2
  Constant4/1 -> Relational Operator/2
  Abs/1 -> Relational Operator/1
  Sum1/1 -> z_pos/1, Data Type Conversion2/1
  z/1 -> Sum1/2
  Demux/1 -> Sum1/1
  x/1 -> Sum2/1
  Demux/2 -> Sum2/2
  Constant3/1 -> Demux/1

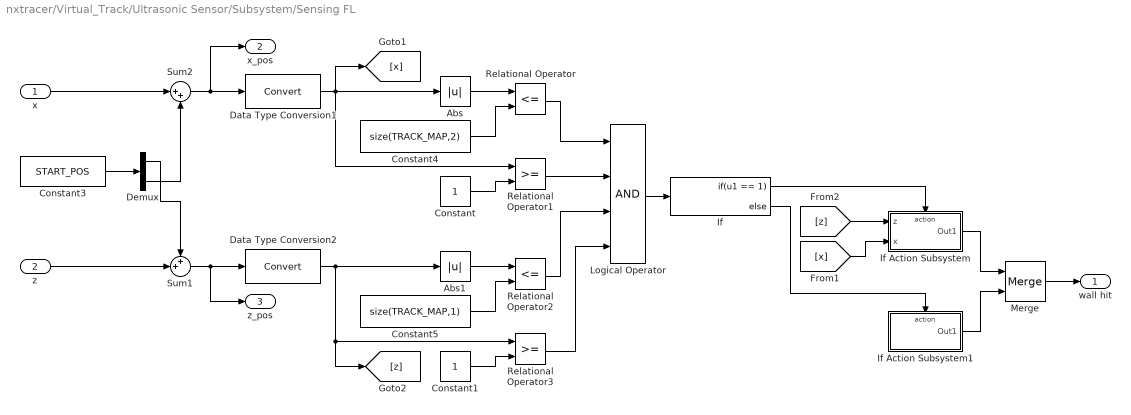
== system nxtracer/Virtual_Track/Ultrasonic Sensor/Subsystem/Sensing FL ==
  x : Inport
  z : Inport  Port=2
  Abs : Abs  SampleTime=-1  SaturateOnIntegerOverflow=off
  Abs1 : Abs  SampleTime=-1  SaturateOnIntegerOverflow=off
  Constant : Constant  Value=1  OutDataType=sfix(16)  ConRadixGroup=Use specified scaling  OutScaling=2^0  SampleTime=inf  FramePeriod=inf
  Constant1 : Constant  Value=1  OutDataType=sfix(16)  ConRadixGroup=Use specified scaling  OutScaling=2^0  SampleTime=inf  FramePeriod=inf
  Constant3 : Constant  Value=START_POS  OutDataType=sfix(16)  ConRadixGroup=Use specified scaling  OutScaling=2^0  SampleTime=inf  FramePeriod=inf
  Constant4 : Constant  Value=size(TRACK_MAP,2)  OutDataType=sfix(16)  ConRadixGroup=Use specified scaling  OutScaling=2^0  SampleTime=inf  FramePeriod=inf
  Constant5 : Constant  Value=size(TRACK_MAP,1)  OutDataType=sfix(16)  ConRadixGroup=Use specified scaling  OutScaling=2^0  SampleTime=inf  FramePeriod=inf
  Data Type Conversion1 : DataTypeConversion  OutDataTypeMode=int32  SaturateOnIntegerOverflow=on
  Data Type Conversion2 : DataTypeConversion  OutDataTypeMode=int32  SaturateOnIntegerOverflow=on
  Demux : Demux  Outputs=2
  If : If  IfExpression=u1 == 1
  If Action Subsystem : Subsystem  TreatAsAtomicUnit=on
  If Action Subsystem1 : Subsystem  TreatAsAtomicUnit=on
  Logical Operator : Logic  Inputs=4  AllPortsSameDT=off  OutDataTypeMode=Boolean
  Merge : Merge
  Relational Operator : RelationalOperator  Operator=<=  LogicOutDataTypeMode=Boolean
  Relational Operator1 : RelationalOperator  LogicOutDataTypeMode=Boolean
  Relational Operator2 : RelationalOperator  Operator=<=  LogicOutDataTypeMode=Boolean
  Relational Operator3 : RelationalOperator  LogicOutDataTypeMode=Boolean
  Sum1 : Sum  Inputs=++|
  Sum2 : Sum  Inputs=|++
  wall hit : Outport
  x_pos : Outport  Port=2
  z_pos : Outport  Port=3
  wires:
  Constant3/1 -> Demux/1
  Demux/2 -> Sum2/2
  x/1 -> Sum2/1
  Demux/1 -> Sum1/1
  z/1 -> Sum1/2
  Sum1/1 -> Data Type Conversion2/1, z_pos/1
  Abs/1 -> Relational Operator/1
  Constant4/1 -> Relational Operator/2
  Constant/1 -> Relational Operator1/2
  Abs1/1 -> Relational Operator2/1
  Constant5/1 -> Relational Operator2/2
  Constant1/1 -> Relational Operator3/2
  Relational Operator/1 -> Logical Operator/1
  Relational Operator2/1 -> Logical Operator/3
  Relational Operator3/1 -> Logical Operator/4
  Logical Operator/1 -> If/1
  Relational Operator1/1 -> Logical Operator/2
  If/1 -> If Action Subsystem/Action
  If/2 -> If Action Subsystem1/Action
  Sum2/1 -> Data Type Conversion1/1, x_pos/1
  Data Type Conversion2/1 -> Abs1/1, Relational Operator3/1, [z]
  Data Type Conversion1/1 -> Abs/1, Relational Operator1/1, [x]
  [z] -> If Action Subsystem/1(z)
  [x] -> If Action Subsystem/2(x)
  If Action Subsystem/1(Out1) -> Merge/1
  If Action Subsystem1/1(Out1) -> Merge/2
  Merge/1 -> wall hit/1

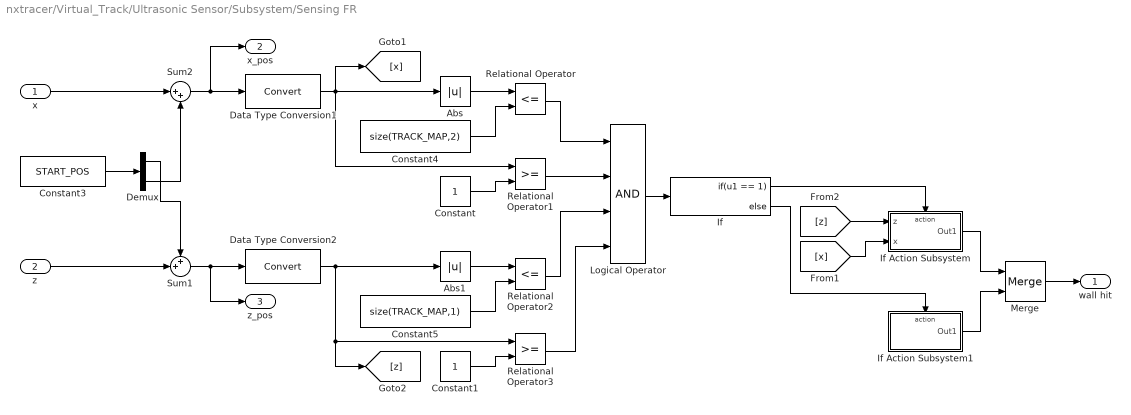
== system nxtracer/Virtual_Track/Ultrasonic Sensor/Subsystem/Sensing FR ==
  x : Inport
  z : Inport  Port=2
  Abs : Abs  SampleTime=-1  SaturateOnIntegerOverflow=off
  Abs1 : Abs  SampleTime=-1  SaturateOnIntegerOverflow=off
  Constant : Constant  Value=1  OutDataType=sfix(16)  ConRadixGroup=Use specified scaling  OutScaling=2^0  SampleTime=inf  FramePeriod=inf
  Constant1 : Constant  Value=1  OutDataType=sfix(16)  ConRadixGroup=Use specified scaling  OutScaling=2^0  SampleTime=inf  FramePeriod=inf
  Constant3 : Constant  Value=START_POS  OutDataType=sfix(16)  ConRadixGroup=Use specified scaling  OutScaling=2^0  SampleTime=inf  FramePeriod=inf
  Constant4 : Constant  Value=size(TRACK_MAP,2)  OutDataType=sfix(16)  ConRadixGroup=Use specified scaling  OutScaling=2^0  SampleTime=inf  FramePeriod=inf
  Constant5 : Constant  Value=size(TRACK_MAP,1)  OutDataType=sfix(16)  ConRadixGroup=Use specified scaling  OutScaling=2^0  SampleTime=inf  FramePeriod=inf
  Data Type Conversion1 : DataTypeConversion  OutDataTypeMode=int32  SaturateOnIntegerOverflow=on
  Data Type Conversion2 : DataTypeConversion  OutDataTypeMode=int32  SaturateOnIntegerOverflow=on
  Demux : Demux  Outputs=2
  If : If  IfExpression=u1 == 1
  If Action Subsystem : Subsystem  TreatAsAtomicUnit=on
  If Action Subsystem1 : Subsystem  TreatAsAtomicUnit=on
  Logical Operator : Logic  Inputs=4  AllPortsSameDT=off  OutDataTypeMode=Boolean
  Merge : Merge
  Relational Operator : RelationalOperator  Operator=<=  LogicOutDataTypeMode=Boolean
  Relational Operator1 : RelationalOperator  LogicOutDataTypeMode=Boolean
  Relational Operator2 : RelationalOperator  Operator=<=  LogicOutDataTypeMode=Boolean
  Relational Operator3 : RelationalOperator  LogicOutDataTypeMode=Boolean
  Sum1 : Sum  Inputs=++|
  Sum2 : Sum  Inputs=|++
  wall hit : Outport
  x_pos : Outport  Port=2
  z_pos : Outport  Port=3
  wires:
  Constant3/1 -> Demux/1
  Demux/2 -> Sum2/2
  x/1 -> Sum2/1
  Demux/1 -> Sum1/1
  z/1 -> Sum1/2
  Sum1/1 -> Data Type Conversion2/1, z_pos/1
  Abs/1 -> Relational Operator/1
  Constant4/1 -> Relational Operator/2
  Constant/1 -> Relational Operator1/2
  Abs1/1 -> Relational Operator2/1
  Constant5/1 -> Relational Operator2/2
  Constant1/1 -> Relational Operator3/2
  Relational Operator/1 -> Logical Operator/1
  Relational Operator2/1 -> Logical Operator/3
  Relational Operator3/1 -> Logical Operator/4
  Logical Operator/1 -> If/1
  Relational Operator1/1 -> Logical Operator/2
  If/1 -> If Action Subsystem/Action
  If/2 -> If Action Subsystem1/Action
  Sum2/1 -> Data Type Conversion1/1, x_pos/1
  Data Type Conversion2/1 -> Abs1/1, Relational Operator3/1, [z]
  Data Type Conversion1/1 -> Abs/1, Relational Operator1/1, [x]
  [z] -> If Action Subsystem/1(z)
  [x] -> If Action Subsystem/2(x)
  If Action Subsystem/1(Out1) -> Merge/1
  If Action Subsystem1/1(Out1) -> Merge/2
  Merge/1 -> wall hit/1

== system nxtracer/Virtual_Track/Virtual Reality/calc camera rot/If Action Subsystem ==
  In1 : Inport
  Action Port : ActionPort  ActionType=then
  Constant1 : Constant  Value=pi  OutDataType=sfix(16)  ConRadixGroup=Use specified scaling  OutScaling=2^0  SampleTime=inf  FramePeriod=inf
  Sum : Sum  Inputs=|+-
  Out1 : Outport
  wires:
  Sum/1 -> Out1/1
  Constant1/1 -> Sum/1
  In1/1 -> Sum/2

== system nxtracer/Virtual_Track/Virtual Reality/calc camera rot/If Action Subsystem1 ==
  In1 : Inport
  Action Port : ActionPort  ActionType=elseif
  Constant1 : Constant  Value=pi  OutDataType=sfix(16)  ConRadixGroup=Use specified scaling  OutScaling=2^0  SampleTime=inf  FramePeriod=inf
  Sum : Sum  Inputs=|-+
  Out1 : Outport
  wires:
  In1/1 -> Sum/2
  Constant1/1 -> Sum/1
  Sum/1 -> Out1/1

== system nxtracer/Virtual_Track/Virtual Reality/calc camera rot/If Action Subsystem2 ==
  In1 : Inport
  Action Port : ActionPort  ActionType=elseif
  Gain : Gain  Gain=-1
  Out1 : Outport
  wires:
  In1/1 -> Gain/1
  Gain/1 -> Out1/1

== system nxtracer/Virtual_Track/Virtual Reality/calc camera rot/If Action Subsystem3 ==
  In1 : Inport
  Action Port : ActionPort  ActionType=else
  Out1 : Outport
  wires:
  In1/1 -> Out1/1

== system nxtracer/Virtual_Track/Virtual Reality/calc rear tyre assy rot/calc rear tyre hub rot ==
  rot : Inport
  speed : Inport  Port=2
  Abs : Abs  SampleTime=-1  SaturateOnIntegerOverflow=off
  Discrete-Time Integrator : DiscreteIntegrator  gainval=1  ExternalReset=falling  InitialConditionSource=external  InitialConditionMode=State only (most efficient)  SampleTime=-1  LimitOutput=on  UpperSaturationLimit=pi/2  LowerSaturationLimit=-pi/2  ICPrevOutput=DiscIntNeverNeededParam  ICPrevScaledInput=DiscIntNeverNeededParam
  Gain2 : Gain  Gain=10
  Gain3 : Gain  Gain=100
  Logical Operator : Logic  Operator=NOT  AllPortsSameDT=off  OutDataTypeMode=Boolean
  Product : Product  RndMeth=Zero
  Relational Operator : RelationalOperator  Operator=>  LogicOutDataTypeMode=Boolean
  Sign : Signum
  Sum : Sum  Inputs=|-+
  Switch : Switch  Threshold=0.5
  Unit Delay : UnitDelay  SampleTime=-1
  Unit Delay1 : UnitDelay  SampleTime=-1
  minimum speed to switch to spining : Constant  Value=0.1  OutDataType=sfix(16)  ConRadixGroup=Use specified scaling  OutScaling=2^0  SampleTime=inf  FramePeriod=inf
  Out1 : Outport
  Out2 : Outport  Port=2
  wires:
  rot/1 -> Sum/1, Unit Delay/1
  Unit Delay/1 -> Sum/2
  Sum/1 -> Gain2/1
  Product/1 -> Unit Delay1/1, Switch/1
  Switch/1 -> Out1/1
  Relational Operator/1 -> Switch/2, Discrete-Time Integrator/2, Logical Operator/1
  minimum speed to switch to spining/1 -> Relational Operator/2
  Logical Operator/1 -> Out2/1
  Sign/1 -> Product/2
  Discrete-Time Integrator/1 -> Switch/3
  Unit Delay1/1 -> Discrete-Time Integrator/3
  Abs/1 -> Relational Operator/1
  speed/1 -> Abs/1, Sign/1
  Gain3/1 -> Discrete-Time Integrator/1
  Gain2/1 -> Gain3/1, Product/1

== system nxtracer/Virtual_Track/Virtual Reality/calc rear tyre assy rot/calc rear tyre rev ==
  spin_flag : Inport
  tyre rotSpeed : Inport  Port=2
  speed : Inport  Port=3
  wall hit : Inport  Port=4
  Abs : Abs  SampleTime=-1  SaturateOnIntegerOverflow=off
  Discrete-Time Integrator1 : DiscreteIntegrator  ExternalReset=level  SampleTime=-1  ICPrevOutput=DiscIntNeverNeededParam  ICPrevScaledInput=DiscIntNeverNeededParam
  Discrete-Time Integrator2 : DiscreteIntegrator  ExternalReset=level  SampleTime=-1  ICPrevOutput=DiscIntNeverNeededParam  ICPrevScaledInput=DiscIntNeverNeededParam
  Gain1 : Gain  Gain=2*pi/(pi*0.02)
  Gain2 : Gain  Gain=W/(pi*0.02)
  Product : Product  RndMeth=Zero
  Selector : Selector  Elements=2  InputPortWidth=2
  Sign : Signum
  Switch : Switch  Threshold=0.5
  Triggered Subsystem : Subsystem  TreatAsAtomicUnit=on
  Unit Delay : UnitDelay  SampleTime=-1
  Out1 : Outport
  wires:
  Switch/1 -> Out1/1
  spin_flag/1 -> Switch/2
  Gain2/1 -> Switch/1
  Gain1/1 -> Switch/3
  speed/1 -> Discrete-Time Integrator2/1
  Discrete-Time Integrator2/1 -> Gain1/1
  tyre rotSpeed/1 -> Selector/1
  Discrete-Time Integrator1/1 -> Abs/1
  wall hit/1 -> Discrete-Time Integrator1/2, Discrete-Time Integrator2/2
  Abs/1 -> Product/2
  Product/1 -> Gain2/1
  Triggered Subsystem/1(Out1) -> Product/1
  Sign/1 -> Triggered Subsystem/Trigger
  Unit Delay/1 -> Sign/1
  Selector/1 -> Discrete-Time Integrator1/1, Unit Delay/1

== system nxtracer/Virtual_Track/Wall hit dection/Wall hit FC/If Action Subsystem ==
  z : Inport
  x : Inport  Port=2
  Action Port : ActionPort  ActionType=then
  Constant1 : Constant  Value=1  OutDataType=sfix(16)  ConRadixGroup=Use specified scaling  OutScaling=2^0  SampleTime=inf  FramePeriod=inf
  Constant5 : Constant  Value=size(TRACK_MAP,1)  OutDataType=sfix(16)  ConRadixGroup=Use specified scaling  OutScaling=2^0  SampleTime=inf  FramePeriod=inf
  Direct Lookup Table (n-D) : simulink/Lookup Tables/Direct Lookup Table (n-D)  maskTabDims=2  explicitNumDims=1  outDims=Element  tabIsInput=off  mxTable=WALL_MAP(:,:,1)  clipFlag=Warning
  Saturation : Saturate  UpperLimit=200  LowerLimit=1
  Saturation1 : Saturate  UpperLimit=200  LowerLimit=1
  Sum1 : Sum  Inputs=-+|
  Sum2 : Sum  Inputs=|+-
  Sum4 : Sum  Inputs=+-|
  Out1 : Outport
  wires:
  Sum4/1 -> Direct Lookup Table (n-D)/1
  Constant5/1 -> Sum4/1
  Saturation/1 -> Sum4/2
  Saturation1/1 -> Direct Lookup Table (n-D)/2
  Sum1/1 -> Saturation1/1
  Sum2/1 -> Saturation/1
  x/1 -> Sum1/2
  Constant1/1 -> Sum1/1, Sum2/2
  z/1 -> Sum2/1
  Direct Lookup Table (n-D)/1 -> Out1/1

== system nxtracer/Virtual_Track/Wall hit dection/Wall hit FC/If Action Subsystem1 ==
  Action Port : ActionPort  ActionType=else
  Constant : Constant  Value=1  OutDataType=sfix(16)  ConRadixGroup=Use specified scaling  OutScaling=2^0  SampleTime=inf  FramePeriod=inf
  Stop Simulation : Stop
  wires:
  Constant/1 -> Stop Simulation/1

== system nxtracer/Virtual_Track/Wall hit dection/Wall hit FL/If Action Subsystem ==
  z : Inport
  x : Inport  Port=2
  Action Port : ActionPort  ActionType=then
  Constant1 : Constant  Value=1  OutDataType=sfix(16)  ConRadixGroup=Use specified scaling  OutScaling=2^0  SampleTime=inf  FramePeriod=inf
  Constant5 : Constant  Value=size(TRACK_MAP,1)  OutDataType=sfix(16)  ConRadixGroup=Use specified scaling  OutScaling=2^0  SampleTime=inf  FramePeriod=inf
  Direct Lookup Table (n-D) : simulink/Lookup Tables/Direct Lookup Table (n-D)  maskTabDims=2  explicitNumDims=1  outDims=Element  tabIsInput=off  mxTable=WALL_MAP(:,:,1)  clipFlag=Warning
  Saturation : Saturate  UpperLimit=200  LowerLimit=1
  Saturation1 : Saturate  UpperLimit=200  LowerLimit=1
  Sum1 : Sum  Inputs=-+|
  Sum2 : Sum  Inputs=|+-
  Sum4 : Sum  Inputs=+-|
  Out1 : Outport
  wires:
  Direct Lookup Table (n-D)/1 -> Out1/1
  z/1 -> Sum2/1
  Constant1/1 -> Sum2/2, Sum1/1
  x/1 -> Sum1/2
  Sum2/1 -> Saturation/1
  Sum1/1 -> Saturation1/1
  Saturation1/1 -> Direct Lookup Table (n-D)/2
  Saturation/1 -> Sum4/2
  Constant5/1 -> Sum4/1
  Sum4/1 -> Direct Lookup Table (n-D)/1

== system nxtracer/Virtual_Track/Wall hit dection/Wall hit FL/If Action Subsystem1 ==
  Action Port : ActionPort  ActionType=else
  Constant : Constant  Value=1  OutDataType=sfix(16)  ConRadixGroup=Use specified scaling  OutScaling=2^0  SampleTime=inf  FramePeriod=inf
  Stop Simulation : Stop
  wires:
  Constant/1 -> Stop Simulation/1

== system nxtracer/Virtual_Track/Wall hit dection/Wall hit FR/If Action Subsystem ==
  z : Inport
  x : Inport  Port=2
  Action Port : ActionPort  ActionType=then
  Constant1 : Constant  Value=1  OutDataType=sfix(16)  ConRadixGroup=Use specified scaling  OutScaling=2^0  SampleTime=inf  FramePeriod=inf
  Constant5 : Constant  Value=size(TRACK_MAP,1)  OutDataType=sfix(16)  ConRadixGroup=Use specified scaling  OutScaling=2^0  SampleTime=inf  FramePeriod=inf
  Direct Lookup Table (n-D) : simulink/Lookup Tables/Direct Lookup Table (n-D)  maskTabDims=2  explicitNumDims=1  outDims=Element  tabIsInput=off  mxTable=WALL_MAP(:,:,1)  clipFlag=Warning
  Saturation : Saturate  UpperLimit=200  LowerLimit=1
  Saturation1 : Saturate  UpperLimit=200  LowerLimit=1
  Sum1 : Sum  Inputs=-+|
  Sum2 : Sum  Inputs=|+-
  Sum4 : Sum  Inputs=+-|
  Out1 : Outport
  wires:
  Direct Lookup Table (n-D)/1 -> Out1/1
  z/1 -> Sum2/1
  Constant1/1 -> Sum2/2, Sum1/1
  x/1 -> Sum1/2
  Sum2/1 -> Saturation/1
  Sum1/1 -> Saturation1/1
  Saturation1/1 -> Direct Lookup Table (n-D)/2
  Saturation/1 -> Sum4/2
  Constant5/1 -> Sum4/1
  Sum4/1 -> Direct Lookup Table (n-D)/1

== system nxtracer/Virtual_Track/Wall hit dection/Wall hit FR/If Action Subsystem1 ==
  Action Port : ActionPort  ActionType=else
  Constant : Constant  Value=1  OutDataType=sfix(16)  ConRadixGroup=Use specified scaling  OutScaling=2^0  SampleTime=inf  FramePeriod=inf
  Stop Simulation : Stop
  wires:
  Constant/1 -> Stop Simulation/1

== system nxtracer/Virtual_Track/Wall hit dection/Wall hit RC/If Action Subsystem ==
  z : Inport
  x : Inport  Port=2
  Action Port : ActionPort  ActionType=then
  Constant1 : Constant  Value=1  OutDataType=sfix(16)  ConRadixGroup=Use specified scaling  OutScaling=2^0  SampleTime=inf  FramePeriod=inf
  Constant5 : Constant  Value=size(TRACK_MAP,1)  OutDataType=sfix(16)  ConRadixGroup=Use specified scaling  OutScaling=2^0  SampleTime=inf  FramePeriod=inf
  Direct Lookup Table (n-D) : simulink/Lookup Tables/Direct Lookup Table (n-D)  maskTabDims=2  explicitNumDims=1  outDims=Element  tabIsInput=off  mxTable=WALL_MAP(:,:,1)  clipFlag=Warning
  Saturation : Saturate  UpperLimit=200  LowerLimit=1
  Saturation1 : Saturate  UpperLimit=200  LowerLimit=1
  Sum1 : Sum  Inputs=-+|
  Sum2 : Sum  Inputs=|+-
  Sum4 : Sum  Inputs=+-|
  Out1 : Outport
  wires:
  Direct Lookup Table (n-D)/1 -> Out1/1
  z/1 -> Sum2/1
  Constant1/1 -> Sum2/2, Sum1/1
  x/1 -> Sum1/2
  Sum2/1 -> Saturation/1
  Sum1/1 -> Saturation1/1
  Saturation1/1 -> Direct Lookup Table (n-D)/2
  Saturation/1 -> Sum4/2
  Constant5/1 -> Sum4/1
  Sum4/1 -> Direct Lookup Table (n-D)/1

== system nxtracer/Virtual_Track/Wall hit dection/Wall hit RC/If Action Subsystem1 ==
  Action Port : ActionPort  ActionType=else
  Constant : Constant  Value=1  OutDataType=sfix(16)  ConRadixGroup=Use specified scaling  OutScaling=2^0  SampleTime=inf  FramePeriod=inf
  Stop Simulation : Stop
  wires:
  Constant/1 -> Stop Simulation/1

== system nxtracer/Virtual_Track/Wall hit dection/Wall hit RL/If Action Subsystem ==
  z : Inport
  x : Inport  Port=2
  Action Port : ActionPort  ActionType=then
  Constant1 : Constant  Value=1  OutDataType=sfix(16)  ConRadixGroup=Use specified scaling  OutScaling=2^0  SampleTime=inf  FramePeriod=inf
  Constant5 : Constant  Value=size(TRACK_MAP,1)  OutDataType=sfix(16)  ConRadixGroup=Use specified scaling  OutScaling=2^0  SampleTime=inf  FramePeriod=inf
  Direct Lookup Table (n-D) : simulink/Lookup Tables/Direct Lookup Table (n-D)  maskTabDims=2  explicitNumDims=1  outDims=Element  tabIsInput=off  mxTable=WALL_MAP(:,:,1)  clipFlag=Warning
  Saturation : Saturate  UpperLimit=200  LowerLimit=1
  Saturation1 : Saturate  UpperLimit=200  LowerLimit=1
  Sum1 : Sum  Inputs=-+|
  Sum2 : Sum  Inputs=|+-
  Sum4 : Sum  Inputs=+-|
  Out1 : Outport
  wires:
  Direct Lookup Table (n-D)/1 -> Out1/1
  z/1 -> Sum2/1
  Constant1/1 -> Sum2/2, Sum1/1
  x/1 -> Sum1/2
  Sum2/1 -> Saturation/1
  Sum1/1 -> Saturation1/1
  Saturation1/1 -> Direct Lookup Table (n-D)/2
  Saturation/1 -> Sum4/2
  Constant5/1 -> Sum4/1
  Sum4/1 -> Direct Lookup Table (n-D)/1

== system nxtracer/Virtual_Track/Wall hit dection/Wall hit RL/If Action Subsystem1 ==
  Action Port : ActionPort  ActionType=else
  Constant : Constant  Value=1  OutDataType=sfix(16)  ConRadixGroup=Use specified scaling  OutScaling=2^0  SampleTime=inf  FramePeriod=inf
  Stop Simulation : Stop
  wires:
  Constant/1 -> Stop Simulation/1

== system nxtracer/Virtual_Track/Wall hit dection/Wall hit RR/If Action Subsystem ==
  z : Inport
  x : Inport  Port=2
  Action Port : ActionPort  ActionType=then
  Constant1 : Constant  Value=1  OutDataType=sfix(16)  ConRadixGroup=Use specified scaling  OutScaling=2^0  SampleTime=inf  FramePeriod=inf
  Constant5 : Constant  Value=size(TRACK_MAP,1)  OutDataType=sfix(16)  ConRadixGroup=Use specified scaling  OutScaling=2^0  SampleTime=inf  FramePeriod=inf
  Direct Lookup Table (n-D) : simulink/Lookup Tables/Direct Lookup Table (n-D)  maskTabDims=2  explicitNumDims=1  outDims=Element  tabIsInput=off  mxTable=WALL_MAP(:,:,1)  clipFlag=Warning
  Saturation : Saturate  UpperLimit=200  LowerLimit=1
  Saturation1 : Saturate  UpperLimit=200  LowerLimit=1
  Sum1 : Sum  Inputs=-+|
  Sum2 : Sum  Inputs=|+-
  Sum4 : Sum  Inputs=+-|
  Out1 : Outport
  wires:
  Sum4/1 -> Direct Lookup Table (n-D)/1
  Constant5/1 -> Sum4/1
  Saturation/1 -> Sum4/2
  Saturation1/1 -> Direct Lookup Table (n-D)/2
  Sum1/1 -> Saturation1/1
  Sum2/1 -> Saturation/1
  x/1 -> Sum1/2
  Constant1/1 -> Sum1/1, Sum2/2
  z/1 -> Sum2/1
  Direct Lookup Table (n-D)/1 -> Out1/1

== system nxtracer/Virtual_Track/Wall hit dection/Wall hit RR/If Action Subsystem1 ==
  Action Port : ActionPort  ActionType=else
  Constant : Constant  Value=1  OutDataType=sfix(16)  ConRadixGroup=Use specified scaling  OutScaling=2^0  SampleTime=inf  FramePeriod=inf
  Stop Simulation : Stop
  wires:
  Constant/1 -> Stop Simulation/1

== system nxtracer/Virtual_Track/Ultrasonic Sensor/Subsystem/Sensing FC/If Action Subsystem ==
  z : Inport
  x : Inport  Port=2
  Action Port : ActionPort  ActionType=then
  Constant1 : Constant  Value=1  OutDataType=sfix(16)  ConRadixGroup=Use specified scaling  OutScaling=2^0  SampleTime=inf  FramePeriod=inf
  Constant5 : Constant  Value=size(TRACK_MAP,1)  OutDataType=sfix(16)  ConRadixGroup=Use specified scaling  OutScaling=2^0  SampleTime=inf  FramePeriod=inf
  Direct Lookup Table (n-D) : simulink/Lookup Tables/Direct Lookup Table (n-D)  maskTabDims=2  explicitNumDims=1  outDims=Element  tabIsInput=off  mxTable=WALL_MAP(:,:,1)  clipFlag=Warning
  Saturation : Saturate  UpperLimit=200  LowerLimit=1
  Saturation1 : Saturate  UpperLimit=200  LowerLimit=1
  Sum1 : Sum  Inputs=-+|
  Sum2 : Sum  Inputs=|+-
  Sum4 : Sum  Inputs=+-|
  Out1 : Outport  InitialOutput=0
  wires:
  Sum4/1 -> Direct Lookup Table (n-D)/1
  Constant5/1 -> Sum4/1
  Saturation/1 -> Sum4/2
  Saturation1/1 -> Direct Lookup Table (n-D)/2
  Sum1/1 -> Saturation1/1
  Sum2/1 -> Saturation/1
  x/1 -> Sum1/2
  Constant1/1 -> Sum1/1, Sum2/2
  z/1 -> Sum2/1
  Direct Lookup Table (n-D)/1 -> Out1/1

== system nxtracer/Virtual_Track/Ultrasonic Sensor/Subsystem/Sensing FC/If Action Subsystem1 ==
  Action Port : ActionPort  ActionType=else
  Constant : Constant  Value=0  OutDataTypeMode=boolean  OutDataType=sfix(16)  ConRadixGroup=Use specified scaling  OutScaling=2^0  SampleTime=inf  FramePeriod=inf
  Out1 : Outport  InitialOutput=0
  wires:
  Constant/1 -> Out1/1

== system nxtracer/Virtual_Track/Ultrasonic Sensor/Subsystem/Sensing FL/If Action Subsystem ==
  z : Inport
  x : Inport  Port=2
  Action Port : ActionPort  ActionType=then
  Constant1 : Constant  Value=1  OutDataType=sfix(16)  ConRadixGroup=Use specified scaling  OutScaling=2^0  SampleTime=inf  FramePeriod=inf
  Constant5 : Constant  Value=size(TRACK_MAP,1)  OutDataType=sfix(16)  ConRadixGroup=Use specified scaling  OutScaling=2^0  SampleTime=inf  FramePeriod=inf
  Direct Lookup Table (n-D) : simulink/Lookup Tables/Direct Lookup Table (n-D)  maskTabDims=2  explicitNumDims=1  outDims=Element  tabIsInput=off  mxTable=WALL_MAP(:,:,1)  clipFlag=Warning
  Saturation : Saturate  UpperLimit=200  LowerLimit=1
  Saturation1 : Saturate  UpperLimit=200  LowerLimit=1
  Sum1 : Sum  Inputs=-+|
  Sum2 : Sum  Inputs=|+-
  Sum4 : Sum  Inputs=+-|
  Out1 : Outport  InitialOutput=0
  wires:
  Direct Lookup Table (n-D)/1 -> Out1/1
  z/1 -> Sum2/1
  Constant1/1 -> Sum2/2, Sum1/1
  x/1 -> Sum1/2
  Sum2/1 -> Saturation/1
  Sum1/1 -> Saturation1/1
  Saturation1/1 -> Direct Lookup Table (n-D)/2
  Saturation/1 -> Sum4/2
  Constant5/1 -> Sum4/1
  Sum4/1 -> Direct Lookup Table (n-D)/1
